simulink model "VSC_GFo_Fixed_Frequency"  (R2015a)
settings: Solver=ode1  SolverMode=SingleTasking  StartTime=0.0  StopTime=2  FixedStep=Time_Step  MaxStep=1e-5  RelTol=1e-3
PreLoadFcn:
  | VSC_GFo_Init;
InitFcn:
  | VSC_GFo_Init;
undefined symbols (not defined in the file): GRD00_Lg, GRD00_Rg, Time_Step, VSC01_Delta_P_Time_Step, VSC01_Delta_P_Value
libraries: powerlib x2, Source_Lib x1, GFo_Lib x1
settings Model: CovMetricSettings=dwe  CovHtmlReporting=off  covSaveCumulativeToWorkspaceVar=off  CovSaveSingleToWorkspaceVar=off  CovExternalEMLEnable=on  Creator=Frederic_Colas  LastModifiedBy=Frederic_Colas
settings DataIOCC: LimitDataPoints=off  SaveFormat=Dataset
settings DebuggingCC: UnconnectedInputMsg=none  UnconnectedOutputMsg=none  UnconnectedLineMsg=none  SFUnexpectedBacktrackingDiag=error  SFNoUnconditionalDefaultTransitionDiag=error
settings HardwareCC: ProdBitPerPointer=64  ProdLargestAtomicFloat=Float  ProdIntDivRoundTo=Zero  ProdEndianess=LittleEndian  ProdHWDeviceType=Specified
settings ModelReferenceCC: PropagateSignalLabelsOutOfModel=on
settings GRTTargetCC: TargetLangStandard=C99 (ISO)  GeneratePreprocessorConditionals=Use local settings
settings SimscapeCC: SimscapeNormalizeSystem=off

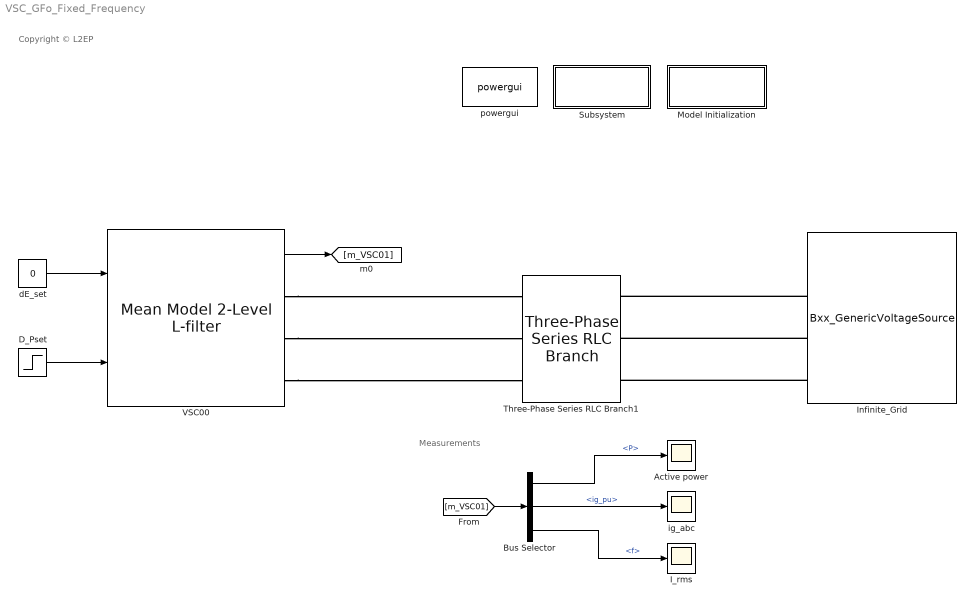
== system VSC_GFo_Fixed_Frequency ==
  note: Copyright © L2EP
  note: Measurements
  Active power : Scope
      settings: TimeRange=auto  LimitDataPoints=on  MaxDataPoints=5000  SaveName=Active_Power  YMin=0.14829  YMax=0.65023  SampleTime=-1  DataFormat=Array  Decimation=10
  Bus Selector : BusSelector  OutputSignals=Control.P,ig_pu,Control.f
  D_Pset : Step  Time=VSC01_Delta_P_Time_Step  After=VSC01_Delta_P_Value  SampleTime=0
  I_rms : Scope
      settings: TimeRange=auto  LimitDataPoints=on  MaxDataPoints=5000  SaveName=ScopeData2  YMin=0.99466  YMax=1.00026  SampleTime=-1  DataFormat=Array  Decimation=10
  Infinite_Grid : Source_Lib/Bxx_GenericVoltageSource  SourceNature_str=INFINITE  fn=50  Sn=1e6  Un=400e3  LFpopup=Swing  P0=-299551241.1925  Q0=4487542.3492  V0_pu=1  U0=20000  Theta0_deg=0  H_s=5  DroopOnOff=on  R_percent=4  TN=1  TD=2
  Model Initialization : Subsystem  mask(Model Functions){InitFcnX=VSC_GFo_Init;, prel=on, posl=off, inif=on, strf=off}
      mask prompts: InitFcnX "Initialisation"; prel "Preload Function"; posl "PostLoad Function"; inif "InitFcn"; strf "StartFcn"
      mask init:
      | currentBlock = gcb;
      | root = bdroot(currentBlock);
      | 
      | if ~strcmp(get_param(root,'BlockDiagramType'),'library')
      |     if prel==1
      |         set_param(root, 'PreLoadFcn', InitFcnX);
      |     else
      |         set_param(root, 'PreLoadFcn', '');
      |     end
      |     if inif==1
      |         set_param(root, 'InitFcn', InitFcnX);
      |     else
      |         set_param(root, 'InitFcn', '');
      |     end
      |     if strf==1
      |         set_param(root, 'StartFcn', InitFcnX);
      |     else
      |         set_param(root, 'StartFcn', '');
      |     end
      |     if posl==1
      |         set_param(root, 'PostLoadFcn', InitFcnX);
      |     else
      |         set_param(root, 'PostLoadFcn', '');
      |     end
      | end
      | 
      | pos = get_param(currentBlock, 'Position');
      | width = pos(3) - pos(1); height = pos(4) - pos(2);
      | txt = [ upper(root) '\n' '- InitFcn. . . . . '  get_param(root, 'InitFcn') ];
      settings: CopyFcn=set_param(gcb,'LinkStatus','none')
      mask Display:
      | %text(5, height*0.5, txt, 'horizontalAlignment', 'left', 'verticalAlignment', 'middle') ;
      | color('blue'),disp('Initialization Function\nParameters')
  Subsystem : Subsystem
      settings: OpenFcn=LoadFlow_VSC
      mask Display: color('blue'),disp('Update Loadflow')
  Three-Phase Series RLC Branch1 : powerlib/Elements/Three-Phase Series RLC Branch  LConnTagsString=A|B|C  RConnTagsString=A|B|C  BranchType=RL  Resistance=GRD00_Rg  Inductance=GRD00_Lg  Capacitance=1e-6  Measurements=None
  VSC00 : GFo_Lib/Mean Model 2-Level L-filter  fn=50  Sn=VSC01_Sn  Pn=VSC01_Pn  Udcn=640e3  Un1=VSC01_Un1  Un2=VSC01_Un2  Rt_pu=VSC01_Rt_pu  Lt_pu=VSC01_Lt_pu  Lm_pu=500  Rm_pu=500  Tr_PLL=VSC01_Tr_PLL  Val_Freq_Support=on  R_percent=VSC01_R  Rv=VSC01_Rv  W_TVR=VSC01_W_LF  I_thresh_pu=VSC01_I_thresh_pu  DX_DR=VSC01_DX_DR  Kp_Rvi_pu=VSC01_Kp_Rvi_pu  gainpopup=1  wc1=VSC01_wc1  mp1=VSC01_mp1  wc2=VSC01_wc2  mp2=VSC01_mp2  wc3=VSC01_wc3  mp3=VSC01_mp3  T1=VSC01_T1  T2=VSC01_T2  LFpopup=PQ  P0=0.3  Q0=1.1858e-08  V0=1.0014  Theta0=0.85828
  dE_set : Constant  Value=0
  ig_abc : Scope
      settings: TimeRange=auto  LimitDataPoints=on  MaxDataPoints=5000  YMin=-2.46712  YMax=2.70682  SampleTime=-1  DataFormat=Array  Decimation=10
  powergui : powerlib/powergui  Priority=1  SimulationMode=Discrete  SampleTime=Time_Step  frequency=60  Iterations=50  frequencyindice=50  Pbase=1000000  ErrMax=1e-4  UnitsV=kV  UnitsW=MW  buscounter=0  FunctionMessages=off  echomessages=off  EnableUseOfTLC=off  CurrentSourceSwitches=off  DisableSnubberDevices=off  DisableRonSwitches=off  DisableVfSwitches=off  DisplayEquations=off  SolverType=Tustin/Backward Euler (TBE)  Interpol=off  ExternalGateDelay=off  methode=off  Ts=100  x0status=blocks  SPID=on  SwTol=0  HookPort=off  RestoreLinks=warning  ResistiveCurrentMeasurement=off  Frange=[0:2:500]  Ylog=off  Xlog=on  ShowGrid=off  save=off  variable=ZData  structure=0  ZoomFFT=off  StartTime=0.0  cycles=1  DisplayStyle=1  fundamental=60  FreqAxis=off  MaxFrequency=1000  frequencyindicesteady=1  RmsSteady=1  display=off
  wires:
  dE_set/1 -> VSC00/1
  D_Pset/1 -> VSC00/2
  [m_VSC01] -> Bus Selector/1
  Bus Selector/1 -> Active power/1  "<P>"
  VSC00/1 -> [m_VSC01]
  Bus Selector/2 -> ig_abc/1  "<ig_pu>"
  Bus Selector/3 -> I_rms/1  "<f>"
  connections:
  VSC00/RConn1 -- Three-Phase Series RLC Branch1/LConn1
  VSC00/RConn3 -- Three-Phase Series RLC Branch1/LConn3
  VSC00/RConn2 -- Three-Phase Series RLC Branch1/LConn2
  Infinite_Grid/RConn1 -- Three-Phase Series RLC Branch1/RConn1
  Infinite_Grid/RConn2 -- Three-Phase Series RLC Branch1/RConn2
  Infinite_Grid/RConn3 -- Three-Phase Series RLC Branch1/RConn3

== system VSC_GFo_Fixed_Frequency/Model Initialization ==

== system VSC_GFo_Fixed_Frequency/Subsystem ==
